simulink model "DinamicaAtuador"  (R2023b)
settings: Solver=FixedStepAuto  StartTime=0.0  StopTime=tf  FixedStep=step_modelo  RelTol=1e-3
undefined symbols (not defined in the file or in its folder): actuator, actuator_nonlin, F_cont_min, Fn, mib, tc, Td, Tpulse
settings Model: Creator=rodri  LastModifiedBy=rodri
settings DataIOCC: SaveOutput=off  SaveTime=off

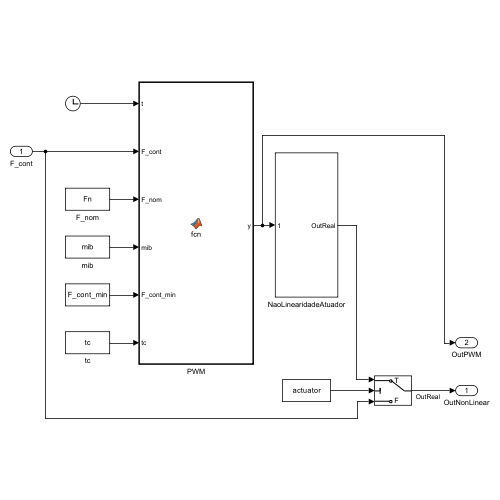
[thumbnail: Simulink's stored preview of the top-level diagram]
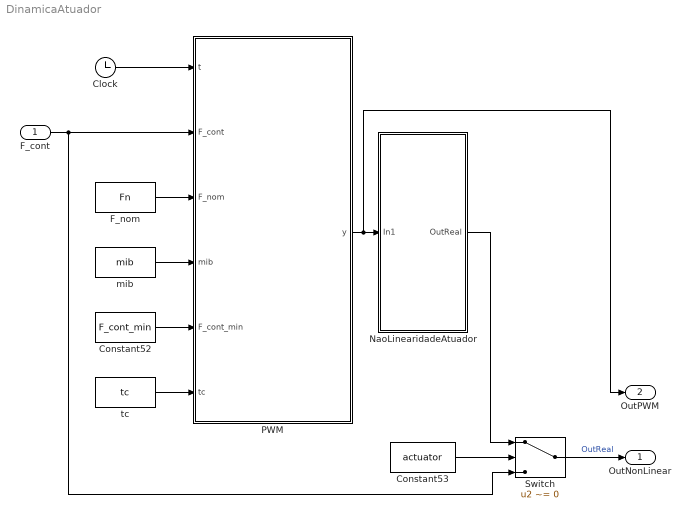
== system DinamicaAtuador ==
  F_cont : Inport  OutDataTypeStr=double  PortDimensions=1
  Clock : Clock
  Constant52 : Constant  Value=F_cont_min  SampleTime=-1
  Constant53 : Constant  Value=actuator  OutDataTypeStr=boolean  SampleTime=-1
  F_nom : Constant  Value=Fn  SampleTime=-1
  NaoLinearidadeAtuador : Subsystem
  PWM : MATLAB Function  TreatAsAtomicUnit=on
  Switch : Switch  Criteria=u2 ~= 0  SaturateOnIntegerOverflow=off  InputSameDT=off
  mib : Constant  Value=mib  SampleTime=-1
  tc : Constant  Value=tc  SampleTime=-1
  OutNonLinear : Outport  OutDataTypeStr=double  PortDimensions=1  SampleTime=0
  OutPWM : Outport  Port=2  OutDataTypeStr=double  PortDimensions=1  SampleTime=0
  wires:
  NaoLinearidadeAtuador/1(OutReal) -> Switch/1
  mib/1 -> PWM/4(mib)
  F_cont/1 -> PWM/2(F_cont), Switch/3
  tc/1 -> PWM/6(tc)
  Constant53/1 -> Switch/2
  F_nom/1 -> PWM/3(F_nom)
  Constant52/1 -> PWM/5(F_cont_min)
  Clock/1 -> PWM/1(t)
  PWM/1(y) -> OutPWM/1, NaoLinearidadeAtuador/1(In1)
  Switch/1 -> OutNonLinear/1  "OutReal"

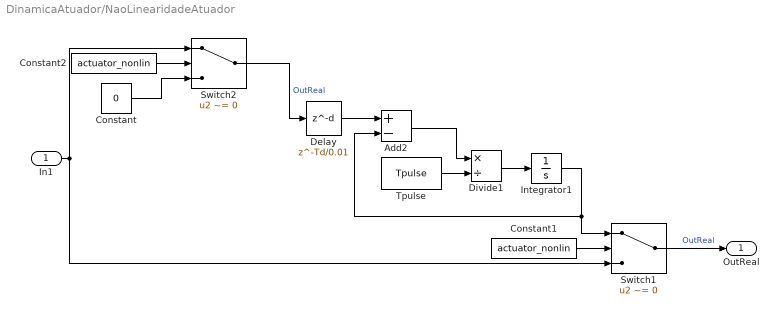
== system DinamicaAtuador/NaoLinearidadeAtuador ==
  In1 : Inport
  Add2 : Sum  Inputs=+-
  Constant : Constant  Value=0
  Constant1 : Constant  Value=actuator_nonlin  OutDataTypeStr=boolean  SampleTime=-1
  Constant2 : Constant  Value=actuator_nonlin  OutDataTypeStr=boolean  SampleTime=-1
  Delay : Delay  DelayLength=Td/0.01  InitialCondition=0
  Divide1 : Product  Inputs=*/
  Integrator1 : Integrator
  Switch1 : Switch  Criteria=u2 ~= 0  SaturateOnIntegerOverflow=off  InputSameDT=off
  Switch2 : Switch  Criteria=u2 ~= 0  SaturateOnIntegerOverflow=off  InputSameDT=off
  Tpulse : Constant  Value=Tpulse  SampleTime=-1
  OutReal : Outport
  wires:
  Switch1/1 -> OutReal/1  "OutReal"
  Constant1/1 -> Switch1/2
  Integrator1/1 -> Switch1/1, Add2/2
  Tpulse/1 -> Divide1/2
  Delay/1 -> Add2/1
  In1/1 -> Switch2/1, Switch1/3
  Add2/1 -> Divide1/1
  Divide1/1 -> Integrator1/1
  Constant2/1 -> Switch2/2
  Switch2/1 -> Delay/1  "OutReal"
  Constant/1 -> Switch2/3

== matlab function DinamicaAtuador/PWM ==
  data: t input; F_cont input; y output; F_nom input; mib input; F_cont_min input; tc input
function y  = fcn(t,F_cont,F_nom,mib,F_cont_min,tc)

if F_cont >= -F_cont_min && F_cont <= F_cont_min
    F_cont = 0;
end

control_cycle = 1/tc;

t_cmd = abs(F_cont)*control_cycle/F_nom; %Tempo de comando (s)

if t_cmd >0 && t_cmd <= mib
    t_cmd = mib;
    pulse_cmd = 100*t_cmd/control_cycle; %porcentagem de atuação (%)
    duty=pulse_cmd;
else
    pulse_cmd = 100*t_cmd/control_cycle; %porcentagem de atuação (%)
    duty=pulse_cmd;
end

if F_cont >= 0
    y = F_nom*square(2*pi*control_cycle.*t,duty);
        if y <= 0
            y = 0;
        end
else
    y = -F_nom*square(2*pi*control_cycle.*t,duty);
        if y >= 0
            y = 0;
        end
end
